simulink model "wilgotnosc"  (R2018b)
settings: Solver=VariableStepAuto  StartTime=0.0  StopTime=intervals  RelTol=1e-3
values from neighbouring files (symbols this model uses):
  intervals = days*stepsInDay    (= 288)    [init.m]
settings Model: Creator=marlon  LastModifiedBy=marlon

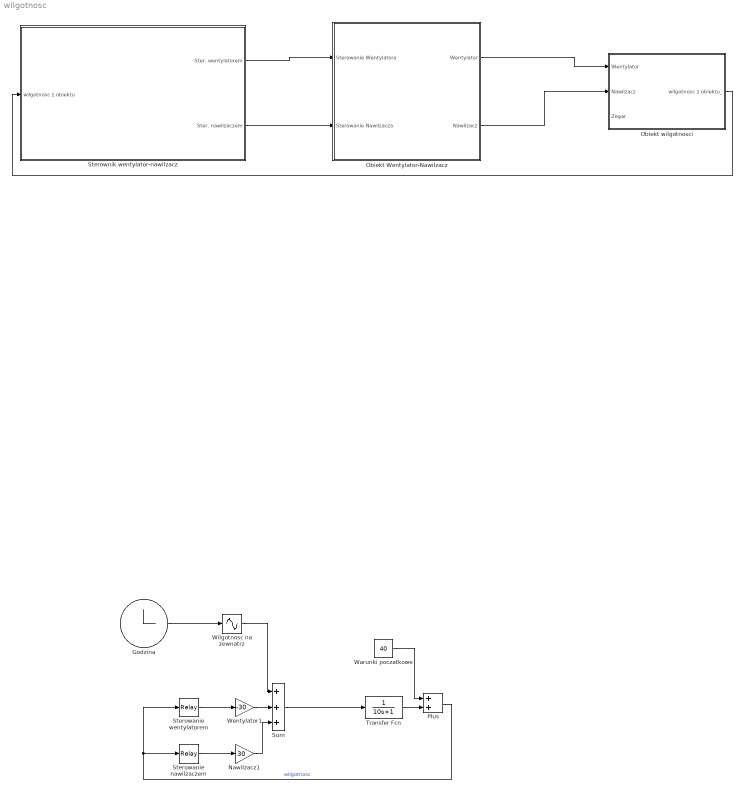
== system wilgotnosc ==
  "Godzina " : Clock
  Nawilzacz1 : Gain  Gain=30
  Obiekt Wentylator-Nawilzacz : Subsystem
  Obiekt wilgotnosci : Subsystem
  Plus : Sum
  Sterowanie nawilzaczem : Relay  OnSwitchValue=60  OffSwitchValue=50  OnOutputValue=0  OffOutputValue=1
  Sterowanie wentylatorem : Relay  OnSwitchValue=70  OffSwitchValue=60
  Sterownik wentylator-nawilzacz : Subsystem
  Sum : Sum  Inputs=+++
  Transfer Fcn : TransferFcn  Denominator=[10 1]
  Warunki poczatkowe : Constant  Value=40
  Wentylator1 : Gain  Gain=-30
  Wilgotnosc na zewnatrz : Sin  TimeSource=Use external signal  Amplitude=20  Bias=20  Frequency=2*pi/intervals  Phase=-pi/2  SampleTime=0
  wires:
  "Godzina "/1 -> Wilgotnosc na zewnatrz/1
  Sum/1 -> Transfer Fcn/1
  Wilgotnosc na zewnatrz/1 -> Sum/1
  Wentylator1/1 -> Sum/2
  Transfer Fcn/1 -> Plus/2
  Sterowanie wentylatorem/1 -> Wentylator1/1
  Plus/1 -> Sterowanie wentylatorem/1, Sterowanie nawilzaczem/1  "wilgotnosc"
  Nawilzacz1/1 -> Sum/3
  Warunki poczatkowe/1 -> Plus/1
  Sterowanie nawilzaczem/1 -> Nawilzacz1/1
  Obiekt Wentylator-Nawilzacz/2(Nawilzacz) -> Obiekt wilgotnosci/2(Nawilzacz)
  Obiekt Wentylator-Nawilzacz/1(Wentylator) -> Obiekt wilgotnosci/1(Wentylator)
  Obiekt wilgotnosci/1(wilgotnosc z obiektu_) -> Sterownik wentylator-nawilzacz/1(wilgotnosc z obiektu)
  Sterownik wentylator-nawilzacz/1(Ster. wentylatorem) -> Obiekt Wentylator-Nawilzacz/1(Sterowanie Wentylatora)
  Sterownik wentylator-nawilzacz/2(Ster. nawilzaczem) -> Obiekt Wentylator-Nawilzacz/2(Sterowanie Nawilzacza)

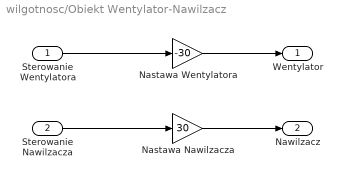
== system wilgotnosc/Obiekt Wentylator-Nawilzacz ==
  Sterowanie Wentylatora : Inport
  Sterowanie Nawilzacza : Inport  Port=2
  Nastawa Nawilzacza : Gain  Gain=30
  Nastawa Wentylatora : Gain  Gain=-30
  Wentylator : Outport
  Nawilzacz : Outport  Port=2
  wires:
  Sterowanie Nawilzacza/1 -> Nastawa Nawilzacza/1
  Sterowanie Wentylatora/1 -> Nastawa Wentylatora/1
  Nastawa Nawilzacza/1 -> Nawilzacz/1
  Nastawa Wentylatora/1 -> Wentylator/1

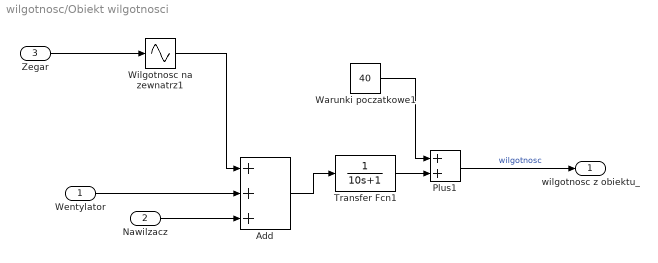
== system wilgotnosc/Obiekt wilgotnosci ==
  Wentylator : Inport
  Nawilzacz : Inport  Port=2
  Zegar : Inport  Port=3
  Add : Sum  Inputs=+++
  Plus1 : Sum
  Transfer Fcn1 : TransferFcn  Denominator=[10 1]
  Warunki poczatkowe1 : Constant  Value=40
  Wilgotnosc na zewnatrz1 : Sin  TimeSource=Use external signal  Amplitude=20  Bias=20  Frequency=2*pi/intervals  Phase=-pi/2  SampleTime=0
  wilgotnosc z obiektu_ : Outport
  wires:
  Wilgotnosc na zewnatrz1/1 -> Add/1
  Plus1/1 -> wilgotnosc z obiektu_/1  "wilgotnosc"
  Nawilzacz/1 -> Add/3
  Add/1 -> Transfer Fcn1/1
  Transfer Fcn1/1 -> Plus1/2
  Zegar/1 -> Wilgotnosc na zewnatrz1/1
  Wentylator/1 -> Add/2
  Warunki poczatkowe1/1 -> Plus1/1

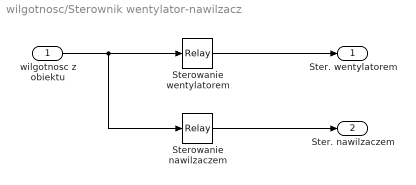
== system wilgotnosc/Sterownik wentylator-nawilzacz ==
  wilgotnosc z obiektu : Inport
  Sterowanie nawilzaczem : Relay  OnSwitchValue=60  OffSwitchValue=50  OnOutputValue=0  OffOutputValue=1
  Sterowanie wentylatorem : Relay  OnSwitchValue=70  OffSwitchValue=60
  Ster. wentylatorem : Outport
  Ster. nawilzaczem : Outport  Port=2
  wires:
  Sterowanie wentylatorem/1 -> Ster. wentylatorem/1
  wilgotnosc z obiektu/1 -> Sterowanie nawilzaczem/1, Sterowanie wentylatorem/1
  Sterowanie nawilzaczem/1 -> Ster. nawilzaczem/1
